simulink model "prueba"  (R2020b)
settings: Solver=VariableStepAuto  StartTime=0.0  StopTime=10.0  RelTol=1e-3
libraries: fuzblock x1
settings Model: Creator=Daniela  LastModifiedBy=Daniela

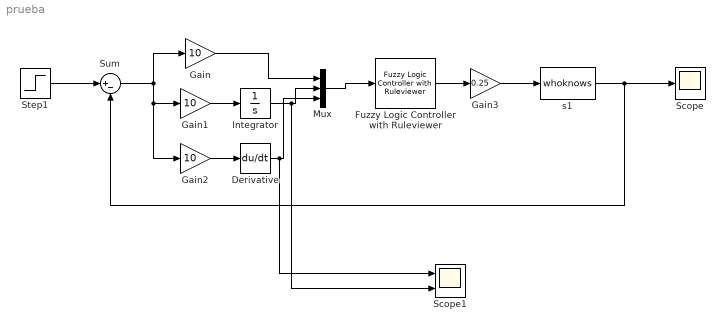
== system prueba ==
  Derivative : Derivative
  Fuzzy Logic Controller with Ruleviewer : fuzblock/Fuzzy Logic  Controller  with Ruleviewer  fismatrix="\"tipper.fis\""  Ts=2
  Gain : Gain  Gain=10
  Gain1 : Gain  Gain=10
  Gain2 : Gain  Gain=10
  Gain3 : Gain  Gain=0.25
  Integrator : Integrator
  Mux : Mux  Inputs=3
  Scope : Scope
  Scope1 : Scope  NumInputPorts=2
  Step1 : Step  SampleTime=0
  Sum : Sum  Inputs=|+-
  s1 : M-S-Function  FunctionName=whoknows  Parameters=L, P1, P2, T, R  mask{L=7, P1=1, P2=7, T=1, R=0}
      mask prompts: L "Laboratorio"; P1 "Primer digito del Puesto"; P2 "Segundo digito del Puesto"; T "Tipo de Planta"; R "Ruido"
      mask Display: disp('Sistema')
  wires:
  Gain3/1 -> s1/1
  Mux/1 -> Fuzzy Logic Controller with Ruleviewer/1
  Fuzzy Logic Controller with Ruleviewer/1 -> Gain3/1
  s1/1 -> Sum/2, Scope/1
  Sum/1 -> Gain1/1, Gain2/1, Gain/1
  Gain2/1 -> Derivative/1
  Derivative/1 -> Scope1/1, Mux/3
  Gain1/1 -> Integrator/1
  Integrator/1 -> Scope1/2, Mux/2
  Gain/1 -> Mux/1
  Step1/1 -> Sum/1
